simulink model "Ejemplo_01_simulink_proceso"  (R2018a)
settings: Solver=VariableStepAuto  StartTime=0.0  StopTime=10.0  RelTol=1e-3
settings Model: Creator=LENOVO  LastModifiedBy=LENOVO

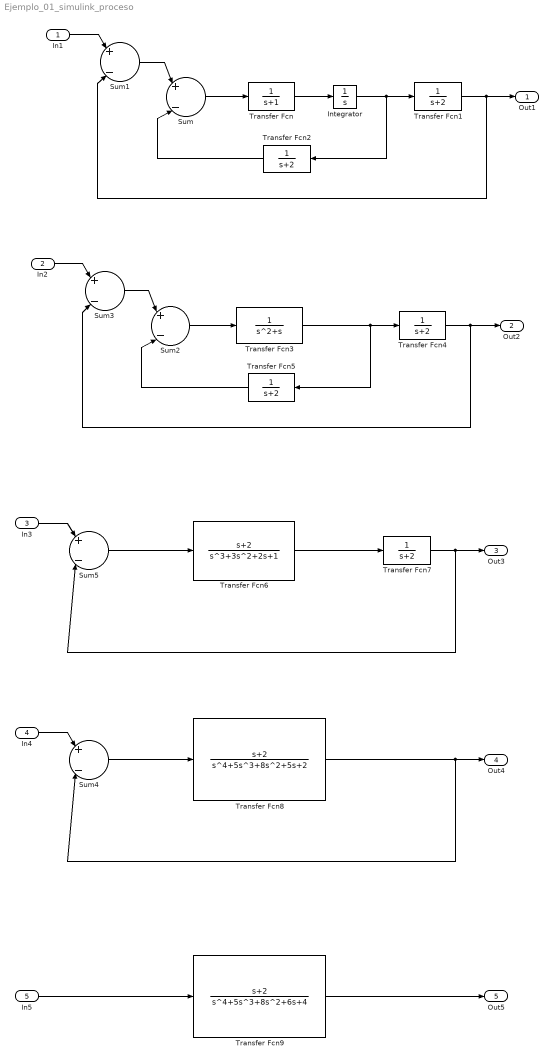
== system Ejemplo_01_simulink_proceso ==
  In1 : Inport
  In2 : Inport  Port=2
  In3 : Inport  Port=3
  In4 : Inport  Port=4
  In5 : Inport  Port=5
  Integrator : Integrator
  Sum{,1..5} (6 alike) : Sum  Inputs=|+|-|
  Transfer Fcn : TransferFcn  Denominator=[1 1]
  Transfer Fcn{1..2,4..5,7} (5 alike) : TransferFcn  Denominator=[1 2]
  Transfer Fcn3 : TransferFcn  Denominator=[1 1 0]
  Transfer Fcn6 : TransferFcn  Numerator=[1 2]  Denominator=[1 3 2 1]
  Transfer Fcn8 : TransferFcn  Numerator=[1 2]  Denominator=[1 5 8 5 2]
  Transfer Fcn9 : TransferFcn  Numerator=[1 2]  Denominator=[1 5 8 6 4]
  Out1 : Outport
  Out2 : Outport  Port=2
  Out3 : Outport  Port=3
  Out4 : Outport  Port=4
  Out5 : Outport  Port=5
  wires:
  Sum/1 -> Transfer Fcn/1
  Transfer Fcn/1 -> Integrator/1
  Integrator/1 -> Transfer Fcn2/1, Transfer Fcn1/1
  Sum1/1 -> Sum/1
  Transfer Fcn2/1 -> Sum/2
  In1/1 -> Sum1/1
  Transfer Fcn1/1 -> Sum1/2, Out1/1
  Transfer Fcn3/1 -> Transfer Fcn5/1, Transfer Fcn4/1
  Transfer Fcn4/1 -> Sum3/2, Out2/1
  Sum3/1 -> Sum2/1
  Transfer Fcn5/1 -> Sum2/2
  Sum2/1 -> Transfer Fcn3/1
  In2/1 -> Sum3/1
  Transfer Fcn6/1 -> Transfer Fcn7/1
  Sum5/1 -> Transfer Fcn6/1
  In3/1 -> Sum5/1
  Transfer Fcn7/1 -> Sum5/2, Out3/1
  Sum4/1 -> Transfer Fcn8/1
  Transfer Fcn8/1 -> Sum4/2, Out4/1
  In4/1 -> Sum4/1
  Transfer Fcn9/1 -> Out5/1
  In5/1 -> Transfer Fcn9/1
